simulink model "Kalman_gefiltert"  (R2019b)
settings: Solver=FixedStepAuto  StartTime=0.0  StopTime=sim  FixedStep=1  RelTol=1e-3
undefined symbols (not defined in the file or in its folder): Discrete, Time
libraries: ctrlSharedLib x1

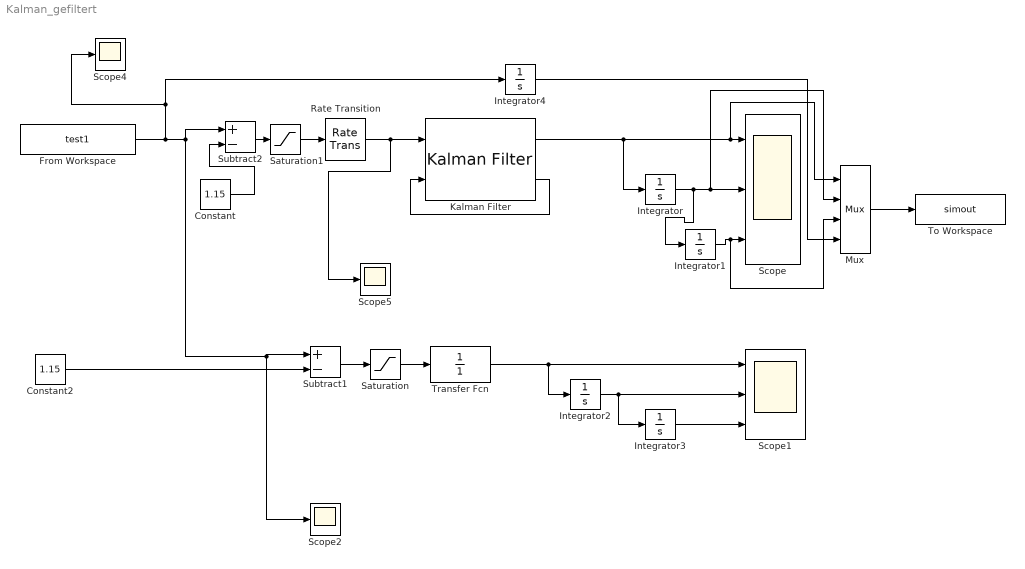
== system Kalman_gefiltert ==
  Constant : Constant  Value=1.15
  Constant2 : Constant  Value=1.15
  From Workspace : FromWorkspace  VariableName=test1  SampleTime=1  Interpolate=off  OutputAfterFinalValue=Setting to zero
  Integrator{,1..4} (5 alike) : Integrator
  Kalman Filter : ctrlSharedLib/Kalman Filter  TimeDomain=Discrete-Time  UseCurrentEstimator=on  ModelSource=LTI State-Space Variable  ModelSourceVariable=ss(0.95,1,1,0,1)  A=0.95  B=1  C=1  D=0  NumberOfStates=1  NumberOfInputs=1  NumberOfOutputs=1  InitialEstimateSource=Dialog  X0=0  P0=10  UseK=off  UseGH=off  NumberOfProcessNoiseInputs=1  G=1  TimeInvariantG=on  H=0  TimeInvariantH=on  Q=0.05  TimeInvariantQ=on  R=1  TimeInvariantR=on  N=0  TimeInvariantN=on  AddInputPort=on  AddEnablePort=off  OutputEstimatedY=on  OutputP=off  Ts=-1
  Mux : Mux
  Rate Transition : RateTransition
  Saturation : Saturate  UpperLimit=inf  LowerLimit=-inf
  Saturation1 : Saturate  UpperLimit=inf  LowerLimit=0
  Scope : Scope  NumInputPorts=3
  Scope1 : Scope  NumInputPorts=3
  Scope2 : Scope
  Scope4 : Scope
  Scope5 : Scope
  Subtract1 : Sum  Inputs=+-
  Subtract2 : Sum  Inputs=+-
  To Workspace : ToWorkspace  VariableName=simout  SaveFormat=Timeseries  SampleTime=-1
  Transfer Fcn : TransferFcn  Denominator=[0 1]
  wires:
  Kalman Filter/2 -> Kalman Filter/2
  Saturation1/1 -> Rate Transition/1
  Kalman Filter/1 -> Integrator/1, Mux/1, Scope/1
  Integrator/1 -> Integrator1/1, Scope/2, Mux/2
  Integrator1/1 -> Mux/3, Scope/3
  Integrator3/1 -> Scope1/3
  Saturation/1 -> Transfer Fcn/1
  Integrator2/1 -> Integrator3/1, Scope1/2
  Subtract1/1 -> Saturation/1
  Subtract2/1 -> Saturation1/1
  Constant2/1 -> Subtract1/2
  From Workspace/1 -> Integrator4/1, Scope4/1, Subtract2/1, Scope2/1, Subtract1/1
  Mux/1 -> To Workspace/1
  Constant/1 -> Subtract2/2
  Integrator4/1 -> Mux/4
  Rate Transition/1 -> Scope5/1, Kalman Filter/1
  Transfer Fcn/1 -> Integrator2/1, Scope1/1
